simulink model "questao2MiguelSimItem4ThamiresPaivaFinal"  (Simulink 8.1)
settings: Solver=ode45  StartTime=0.0  StopTime=100  MaxStep=0.01  RelTol=1e-3
values from neighbouring files (symbols this model uses):
  A = [0 1  0              0 ... (first row only)    [MatLab4p.m]    (also in MatLab5p.m = [     0        1       0        0; MatLab6p_solucao4.m = [     0        1       0        0; MatLab7p.m = [0 1; -5*sqrt(2) -1]; pplane8.m = [)
  Am = blkdiag(M,M)    [MatLab5p.m]    (also in MatLab6p_solucao4.m; questao2Miguel.m = blkdiag(M); questao2MiguelFinal.m = blkdiag(M))
  Am2 = blkdiag(M)    [questao2Miguel.m]    (also in questao2MiguelFinal.m)
  B = [0; 1/M; 0; -1/(M*L)]    [MatLab4p.m]    (also in MatLab5p.m = [ 0    0; MatLab6p_solucao4.m = [ 0    0; MatLab7p.m = [0 ; 10]; pplane8.m = real(A))
  Bm = blkdiag(N,N)    [MatLab5p.m]    (also in MatLab6p_solucao4.m; questao2Miguel.m = blkdiag(N); questao2MiguelFinal.m = blkdiag(N))
  Bm2 = blkdiag(N)    [questao2Miguel.m]    (also in questao2MiguelFinal.m)
  C = [1 0 0 0]    [MatLab4p.m]    (also in MatLab5p.m = [1 0 0 0; MatLab6p_solucao4.m = [1 0 0 0; MatLab7p.m = [1 0]; pplane8.m = imag(A))
  Dsim = zeros(4,1)    [MatLab4p.m]    (also in MatLab5p.m = zeros(4,2); MatLab6p_solucao4.m = zeros(4,2); questao2Miguel.m; questao2MiguelFinal.m)
  K = place(A,B,[-3 -3.05 -3.1 -3.15])    [MatLab4p.m]    (also in MatLab5p.m = Ka(:,1:4); MatLab6p_solucao4.m = Ka(:,1:4); MatLab7p.m = place(A,B,[-4 -4.05]); pplane8.m = kk +2*(jj-1))
  K2 = Ka2(1:4)    [questao2Miguel.m]    (also in questao2MiguelFinal.m)
  Km = Ka(:,5:10)    [MatLab5p.m]    (also in MatLab6p_solucao4.m = Ka(:,5:12); MatLab7p.m = Ka(1,3); questao2Miguel.m = Ka(5); questao2MiguelFinal.m = Ka(5))
  Km2 = Ka2(5:6)    [questao2Miguel.m]    (also in questao2MiguelFinal.m)
  Lobs = H'    [MatLab6p_solucao4.m]    (also in questao2Miguel.m; questao2MiguelFinal.m)
  x0 = [0 0 pi/4 0]    [MatLab4p.m]    (also in MatLab5p.m = [1 0.5 1 0.1]; MatLab6p_solucao4.m = [0 0 0 0]; MatLab7p.m = [0 ; 0]; questao2Miguel.m = [0 0.01 0.3 0])
  x0obs = [0 0 0 0]    [MatLab4p.m]    (also in MatLab6p_solucao4.m; MatLab7p.m = [0 ; 0]; questao2Miguel.m; questao2MiguelFinal.m)
settings Model: Creator=hector  LastModifiedBy=Deinis-UFSC
settings DataIOCC: SignalLoggingSaveFormat=Dataset
settings OptimizationCC: ExpressionDepthLimit=128
settings DebuggingCC: UnderspecifiedInitializationDetection=Simplified  MergeDetectMultiDrivingBlocksExec=error  FcnCallInpInsideContextMsg=EnableAllAsError  FrameProcessingCompatibilityMsg=error  StateNameClashWarn=none
settings GRTTargetCC: CodeReplacementLibrary=C89/C90 (ANSI)  CombineOutputUpdateFcns=on  GRTInterface=off

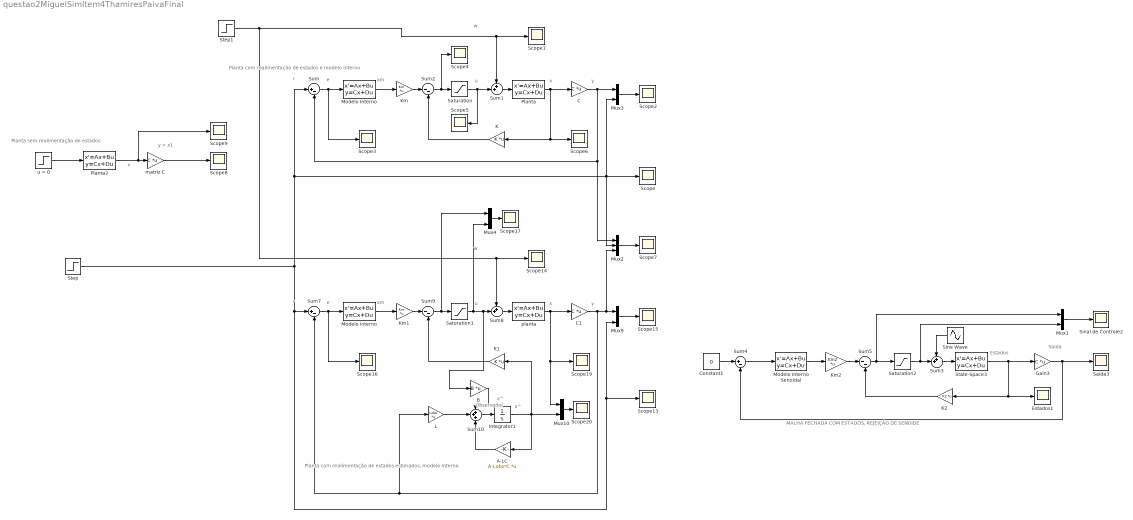
== system questao2MiguelSimItem4ThamiresPaivaFinal ==
  note: Planta com realimentação de estados estimados, modelo interno
  note: Planta com realimentação de estados e modelo interno
  note: w
  note: u
  note: xm
  note: e
  note: r
  note: x
  note: y
  note: w
  note: u
  note: xm
  note: e
  note: r
  note: x
  note: y
  note: Observador
  note: x^
  note: x^
  note: Planta sem realimentação de estados
  note: x
  note: y = x1
  note: MALHA FECHADA COM ESTADOS, REJEIÇÃO DE SENOIDE
  note: Saida
  note: Estados
  A-LC : Gain  Gain=A-Lobs*C  Multiplication=Matrix(K*u)
  B : Gain  Gain=B  Multiplication=Matrix(K*u)
  C : Gain  Gain=C  Multiplication=Matrix(K*u)
  C1 : Gain  Gain=C  Multiplication=Matrix(K*u)
  Constant1 : Constant  Value=0
  Estados1 : Scope
      settings: TimeRange=auto  LimitDataPoints=on  MaxDataPoints=5000  SaveToWorkspace=off  SaveName=ScopeData3  YMin=-10  YMax=10  SampleTime=-1  DataFormat=Array
  Gain3 : Gain  Gain=C  Multiplication=Matrix(K*u)
  Integrator1 : Integrator  InitialCondition=x0obs
  K : Gain  Gain=K  Multiplication=Matrix(K*u)
  K1 : Gain  Gain=K  Multiplication=Matrix(K*u)
  K2 : Gain  Gain=K2  Multiplication=Matrix(K*u)
  Km : Gain  Gain=Km  Multiplication=Matrix(K*u)
  Km1 : Gain  Gain=Km  Multiplication=Matrix(K*u)
  Km2 : Gain  Gain=Km2  Multiplication=Matrix(K*u)
  L : Gain  Gain=Lobs  Multiplication=Matrix(K*u)
  Modelo Interno : StateSpace  A=Am  B=Bm  D=0  X0=0
  Modelo Interno Senoidal : StateSpace  A=Am2  B=Bm2  C=eye(2)  D=zeros(2, 1)  X0=0
  Modelo interno : StateSpace  A=Am  B=Bm  D=0  X0=0
  Mux{1,3..4,9..10} (5 alike) : Mux  Inputs=2
  Mux2 : Mux  Inputs=3
  Planta : StateSpace  A=A  B=B  C=eye(4)  D=Dsim  X0=x0
  Planta2 : StateSpace  A=A  B=B  C=eye(4)  D=Dsim  X0=x0
  Saida3 : Scope
      settings: TimeRange=auto  MaxDataPoints=5000  SaveToWorkspace=off  SaveName=ScopeData4  YMin=-0.10657  YMax=0.06587  SampleTime=-1  DataFormat=Array
  Saturation : Saturate  UpperLimit=20  LowerLimit=-20
  Saturation1 : Saturate  UpperLimit=50  LowerLimit=-50
  Saturation2 : Saturate  UpperLimit=50  LowerLimit=-50
  Scope{,1..9,13..17,19..20} (17 alike) : Scope
      Scope settings: TimeRange=auto  MaxDataPoints=5000  SaveToWorkspace=off  SaveName=ScopeData  YMin=-10  YMax=10  SampleTime=-1  DataFormat=Array
      Scope1 settings: TimeRange=auto  MaxDataPoints=5000  SaveToWorkspace=off  YMin=-10  YMax=10  SampleTime=-1  DataFormat=Array
      Scope13 settings: TimeRange=auto  MaxDataPoints=5000  SaveToWorkspace=off  SaveName=ScopeData13  YMin=-10  YMax=10  SampleTime=-1  DataFormat=Array
      Scope14 settings: TimeRange=auto  MaxDataPoints=5000  SaveToWorkspace=off  SaveName=ScopeData14  YMin=-10  YMax=10  SampleTime=-1  DataFormat=Array
      Scope15 settings: TimeRange=auto  MaxDataPoints=5000  SaveToWorkspace=off  SaveName=ScopeData15  YMin=-1.91177  YMax=2.21111  SampleTime=-1  DataFormat=Array
      Scope16 settings: TimeRange=auto  MaxDataPoints=5000  SaveToWorkspace=off  SaveName=ScopeData16  YMin=-0.035  YMax=0.0025  SampleTime=-1  DataFormat=Array
      Scope17 settings: TimeRange=auto  MaxDataPoints=5000  SaveToWorkspace=off  SaveName=ScopeData17  YMin=-181.98355  YMax=143.3644  SampleTime=-1  DataFormat=Array
      Scope19 settings: TimeRange=auto  ShowLegends=on  LimitDataPoints=on  MaxDataPoints=5000  SaveToWorkspace=off  SaveName=ScopeData19  YMin=-0.5  YMax=3.25  SampleTime=-1
      Scope2 settings: TimeRange=auto  MaxDataPoints=5000  SaveToWorkspace=off  SaveName=ScopeData2  YMin=1.9  YMax=3.3  SampleTime=-1  DataFormat=Array
      Scope20 settings: TimeRange=auto  ShowLegends=on  MaxDataPoints=5000  SaveToWorkspace=off  SaveName=ScopeData20  YMin=-1.5  YMax=3.25  SampleTime=-1  DataFormat=Array
      Scope3 settings: TimeRange=auto  MaxDataPoints=5000  SaveToWorkspace=off  SaveName=ScopeData3  YMin=-0.035  YMax=0.0025  SampleTime=-1  DataFormat=Array
      Scope4 settings: TimeRange=auto  MaxDataPoints=5000  SaveToWorkspace=off  SaveName=ScopeData4  YMin=-2.5  YMax=50  SampleTime=-1  DataFormat=Array
      Scope5 settings: TimeRange=auto  MaxDataPoints=5000  SaveToWorkspace=off  SaveName=ScopeData5  YMin=1  YMax=6  SampleTime=-1  DataFormat=Array
      Scope6 settings: TimeRange=auto  ShowLegends=on  LimitDataPoints=on  MaxDataPoints=5000  SaveToWorkspace=off  SaveName=ScopeData6  YMin=-0.5  YMax=3.25  SampleTime=-1
      Scope7 settings: TimeRange=auto  ShowLegends=on  MaxDataPoints=5000  SaveToWorkspace=off  SaveName=ScopeData7  YMin=-0.92844  YMax=1.95406  SampleTime=-1  DataFormat=Array
      Scope8 settings: TimeRange=auto  MaxDataPoints=5000  SaveToWorkspace=off  YMin=-73952566909512330000000000000000000000000000000000000000000000000000000000000000000000000000000000000000000000000000000000000000000000000000000000000000000000000000.00000  YMax=8216951878834702500000000000000000000000000000000000000000000000000000000000000000000000000000000000000000000000000000000000000000000000000000000000000000000000000.00000  SampleTime=-1
      Scope9 settings: TimeRange=auto  MaxDataPoints=5000  SaveToWorkspace=off  SaveName=ScopeData2  YMin=-378244065531178270000000000000000000000000000000000000000000000000000000000000000000000000000000000000000000000000000000000000000000000000000000000000000000000000000.00000  YMax=882569486239415910000000000000000000000000000000000000000000000000000000000000000000000000000000000000000000000000000000000000000000000000000000000000000000000000000.00000  SampleTime=-1
  Sinal de Controle2 : Scope
      settings: TimeRange=auto  MaxDataPoints=5000  SaveToWorkspace=off  SaveName=ScopeData5  YMin=-6.25085  YMax=6.25085  SampleTime=-1  DataFormat=Array
  Sine Wave : Sin  Amplitude=5  Frequency=0.1  SampleTime=0
  State-Space3 : StateSpace  A=A  B=B  C=eye(4)  D=Dsim  X0=x0
  Step : Step  Time=0  SampleTime=0
  Step1 : Step  Time=15  After=0.5  SampleTime=0
  Sum : Sum  Inputs=|+-
  Sum1 : Sum  Inputs=++|
  Sum10 : Sum  Inputs=+++
  Sum2 : Sum  Inputs=|--
  Sum3 : Sum  Inputs=++|
  Sum4 : Sum  Inputs=|+-
  Sum5 : Sum  Inputs=|--
  Sum7 : Sum  Inputs=|+-
  Sum8 : Sum  Inputs=++|
  Sum9 : Sum  Inputs=|--
  matriz C : Gain  Gain=C  Multiplication=Matrix(K*u)
  planta : StateSpace  A=A  B=B  C=eye(4)  D=Dsim  X0=x0
  "u = 0 " : Step  Time=0  After=0  SampleTime=0
  wires:
  Sum/1 -> Modelo Interno/1, Scope3/1
  Sum1/1 -> Planta/1
  Planta/1 -> C/1, Scope6/1, K/1
  Mux3/1 -> Scope2/1
  Sum2/1 -> Saturation/1, Scope4/1
  Km/1 -> Sum2/1
  Modelo Interno/1 -> Km/1
  K/1 -> Sum2/2
  C/1 -> Mux3/1, Sum/2, Mux2/1
  Step/1 -> Sum/1, Mux2/2, Scope/1, Mux3/2, Sum7/1, Scope13/1, Mux9/2
  Saturation/1 -> Sum1/2, Scope5/1
  Sum7/1 -> Modelo interno/1, Scope16/1
  Sum8/1 -> planta/1
  Step1/1 -> Sum8/1, Scope14/1, Sum1/1, Scope1/1
  planta/1 -> C1/1, Scope19/1, Mux10/1
  Mux9/1 -> Scope15/1
  Sum9/1 -> Mux4/1, Saturation1/1
  Km1/1 -> Sum9/1
  Modelo interno/1 -> Km1/1
  K1/1 -> Sum9/2
  C1/1 -> Mux2/3, Mux9/1, L/1, Sum7/2
  Saturation1/1 -> Mux4/2, B/1, Sum8/2
  Sum10/1 -> Integrator1/1
  L/1 -> Sum10/2
  A-LC/1 -> Sum10/3
  Integrator1/1 -> Mux10/2, A-LC/1, K1/1
  B/1 -> Sum10/1
  Mux10/1 -> Scope20/1
  Mux2/1 -> Scope7/1
  "u = 0 "/1 -> Planta2/1
  matriz C/1 -> Scope8/1
  Planta2/1 -> Scope9/1, matriz C/1
  State-Space3/1 -> Gain3/1, K2/1, Estados1/1
  Gain3/1 -> Sum4/2, Saida3/1
  Sum4/1 -> Modelo Interno Senoidal/1
  Modelo Interno Senoidal/1 -> Km2/1
  Km2/1 -> Sum5/1
  K2/1 -> Sum5/2
  Sum3/1 -> State-Space3/1
  Sine Wave/1 -> Sum3/1
  Sum5/1 -> Saturation2/1, Mux1/1
  Saturation2/1 -> Sum3/2, Mux1/2
  Mux1/1 -> Sinal de Controle2/1
  Constant1/1 -> Sum4/1
  Mux4/1 -> Scope17/1
